simulink model "csss_22"  (R2020b)
settings: Solver=VariableStepAuto  StartTime=0.0  StopTime=10  RelTol=1e-3
settings Model: Creator=win10  LastModifiedBy=win10

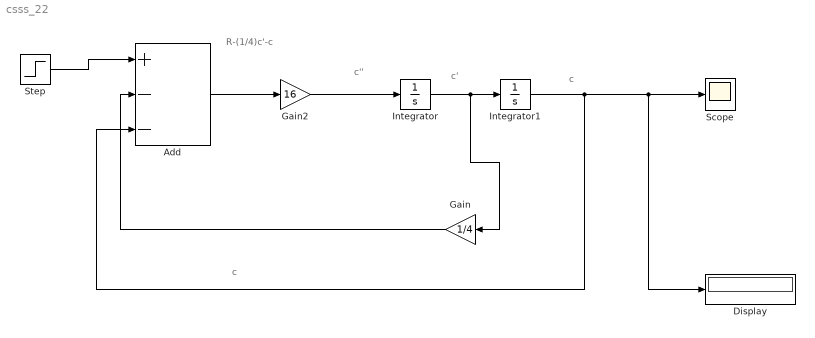
== system csss_22 ==
  note: c
  note: R-(1/4)c'-c
  note: c
  note: c'
  note: c''
  Add : Sum  Inputs=+--
  Display : Display
  Gain : Gain  Gain=1/4
  Gain2 : Gain  Gain=16
  Integrator : Integrator
  Integrator1 : Integrator
  Scope : Scope
  Step : Step  SampleTime=0
  wires:
  Step/1 -> Add/1
  Add/1 -> Gain2/1
  Integrator/1 -> Gain/1, Integrator1/1
  Gain/1 -> Add/2
  Integrator1/1 -> Add/3, Display/1, Scope/1
  Gain2/1 -> Integrator/1
